simulink model "Task_2"  (R2023b)
settings: Solver=VariableStepAuto  StartTime=0.0  StopTime=10.0  RelTol=1e-3
StopFcn:
  | subplot(2,1,1)
  | plot(out.Output);
  | xlabel('Time Seconds')
  | ylabel('Amplitude')
  | title('First Output')
  | 
  | subplot(2,1,2)
  | plot(out.Output1);
  | xlabel('Time Seconds')
  | ylabel('Amplitude')
  | title('First Output')
settings Model: Creator=Azlaan  LastModifiedBy=Azlaan

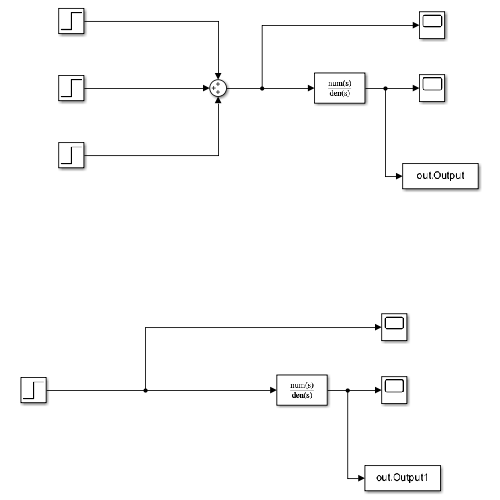
[thumbnail: Simulink's stored preview of the top-level diagram]
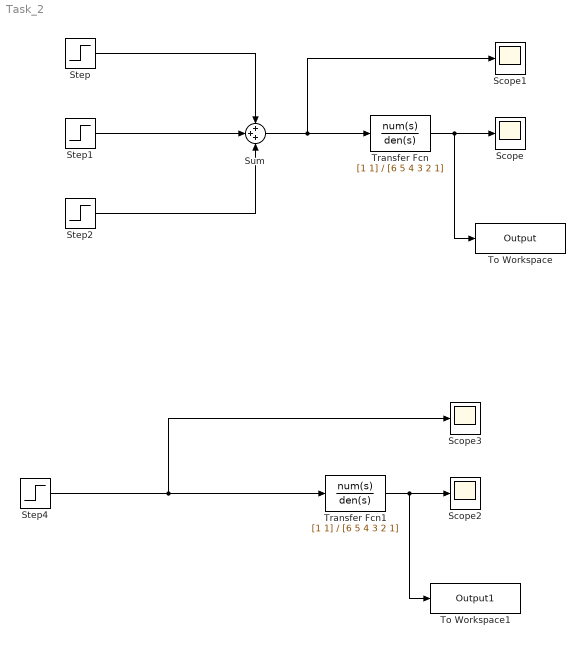
== system Task_2 ==
  Scope{,1..3} (4 alike) : Scope
  Step{,1..2,4} (4 alike) : Step  SampleTime=0
  Sum : Sum  Inputs=+++
  To Workspace : ToWorkspace  VariableName=Output  SaveFormat=Timeseries  SampleTime=-1
  To Workspace1 : ToWorkspace  VariableName=Output1  SaveFormat=Timeseries  SampleTime=-1
  Transfer Fcn : TransferFcn  Numerator=[1 1]  Denominator=[6 5 4 3 2 1]
  Transfer Fcn1 : TransferFcn  Numerator=[1 1]  Denominator=[6 5 4 3 2 1]
  wires:
  Step/1 -> Sum/1
  Step1/1 -> Sum/2
  Step2/1 -> Sum/3
  Sum/1 -> Scope1/1, Transfer Fcn/1
  Transfer Fcn/1 -> To Workspace/1, Scope/1
  Transfer Fcn1/1 -> To Workspace1/1, Scope2/1
  Step4/1 -> Scope3/1, Transfer Fcn1/1
